simulink model "SMC_Altitude_PID_Position"  (R2021a)
settings: Solver=VariableStepAuto  StartTime=0.0  StopTime=20  RelTol=1e-3
InitFcn:
  | run Quadcopter_setup_parameters.m
values from neighbouring files (symbols this model uses):
  b = 0.001    [Quadcopter_setup_parameters.m]
  Dx = 0.1    [Quadcopter_setup_parameters.m]
  Dy = Dx    (= 0.1)    [Quadcopter_setup_parameters.m]
  Dz = Dx    (= 0.1)    [Quadcopter_setup_parameters.m]
  g = 9.81    [Quadcopter_setup_parameters.m]    (also in recording.mat = 9.80665; uas_parameters.m = 9.80665; uas_parameters.mat = 9.80665)
  I = diag([Ixx; Iyy;Izz],0)    [Quadcopter_setup_parameters.m]
  k = 0.01    [Quadcopter_setup_parameters.m]
  k_phi = 10    [Quadcopter_setup_parameters.m]
  k_psi = 10    [Quadcopter_setup_parameters.m]
  k_theta = 10    [Quadcopter_setup_parameters.m]
  k_z = 10    [Quadcopter_setup_parameters.m]
  kd_xy = 1    [Quadcopter_setup_parameters.m]
  kp_xy = 1    [Quadcopter_setup_parameters.m]
  L = 0.225    [Quadcopter_setup_parameters.m]
  lambda_phi = 2    [Quadcopter_setup_parameters.m]
  lambda_psi = 2    [Quadcopter_setup_parameters.m]
  lambda_theta = 2    [Quadcopter_setup_parameters.m]
  lambda_z = 2    [Quadcopter_setup_parameters.m]
  m = 0.55    [Quadcopter_setup_parameters.m]
settings Model: Creator=Kristian  LastModifiedBy=dwuth
settings SolverCC: AlgebraicLoopSolver=TrustRegion
settings DebuggingCC: SFMachineParentedDataDiag=warning

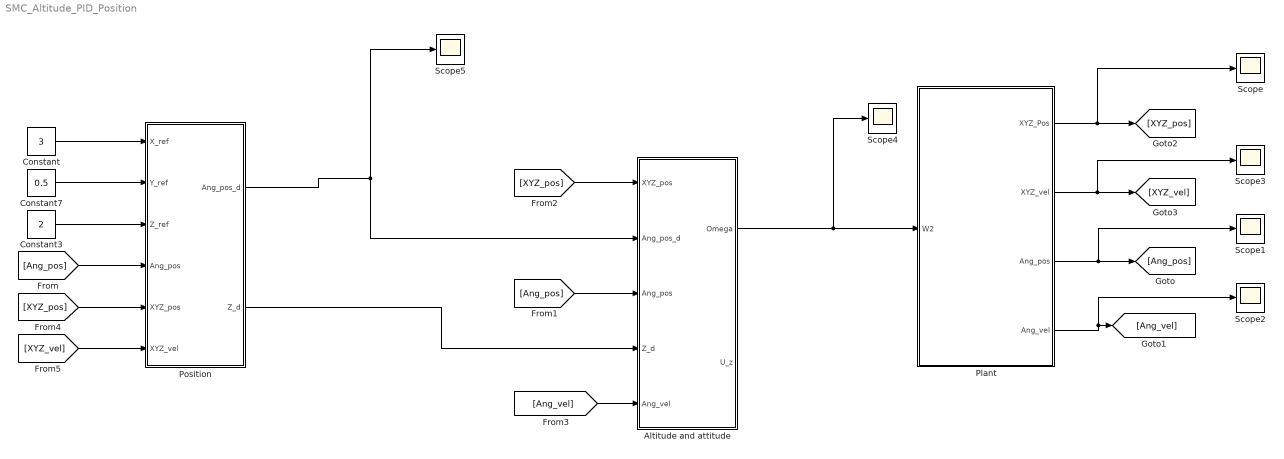
== system SMC_Altitude_PID_Position ==
  Altitude and attitude : Subsystem
  Constant : Constant  Value=3
  Constant3 : Constant  Value=2
  Constant7 : Constant  Value=0.5
  Plant : Subsystem
  Position : Subsystem
  Scope{,1..5} (6 alike) : Scope
  wires:
  Plant/3(Ang_pos) -> [Ang_pos], Scope1/1
  Plant/1(XYZ_Pos) -> [XYZ_pos], Scope/1
  Plant/4(Ang_vel) -> [Ang_vel], Scope2/1
  Altitude and attitude/1(Omega) -> Scope4/1, Plant/1(W2)
  [Ang_vel] -> Altitude and attitude/5(Ang_vel)
  [Ang_pos] -> Altitude and attitude/3(Ang_pos)
  [XYZ_pos] -> Altitude and attitude/1(XYZ_pos)
  Plant/2(XYZ_vel) -> Scope3/1, [XYZ_vel]
  [Ang_pos] -> Position/4(Ang_pos)
  Constant/1 -> Position/1(X_ref)
  Constant7/1 -> Position/2(Y_ref)
  [XYZ_pos] -> Position/5(XYZ_pos)
  [XYZ_vel] -> Position/6(XYZ_vel)
  Position/1(Ang_pos_d) -> Altitude and attitude/2(Ang_pos_d), Scope5/1
  Constant3/1 -> Position/3(Z_ref)
  Position/2(Z_d) -> Altitude and attitude/4(Z_d)

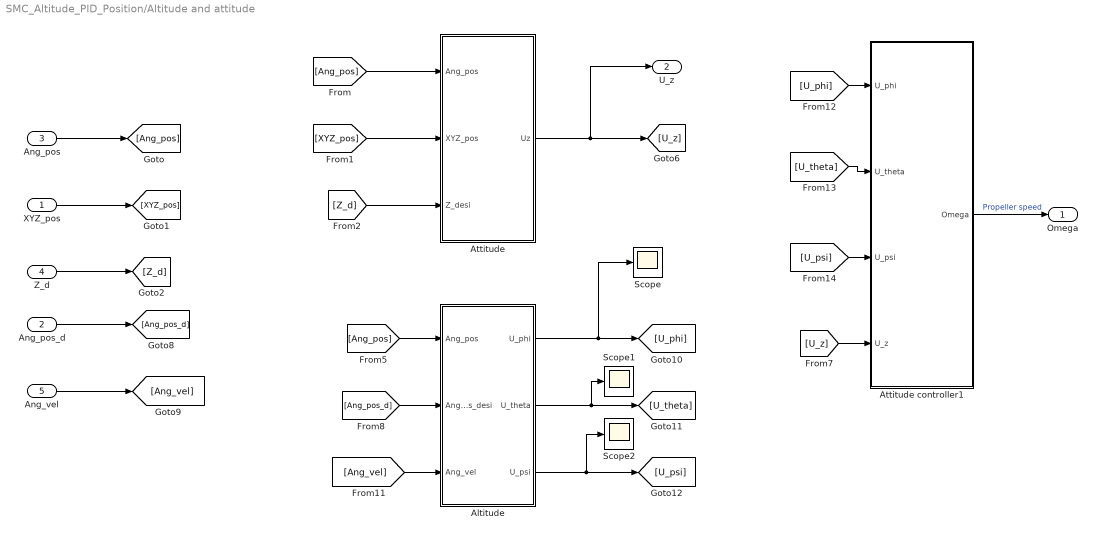
== system SMC_Altitude_PID_Position/Altitude and attitude ==
  XYZ_pos : Inport
  Ang_pos_d : Inport  Port=2
  Ang_pos : Inport  Port=3
  Z_d : Inport  Port=4
  Ang_vel : Inport  Port=5
  Altitude : Subsystem
  Attitude : Subsystem
  Attitude controller1 : MATLAB Function  TreatAsAtomicUnit=on
  Scope : Scope
  Scope1 : Scope
  Scope2 : Scope
  Omega : Outport
  U_z : Outport  Port=2
  wires:
  Attitude controller1/1(Omega) -> Omega/1  "Propeller speed"
  Z_d/1 -> [Z_d]
  [U_theta] -> Attitude controller1/2(U_theta)
  Ang_pos_d/1 -> [Ang_pos_d]
  [XYZ_pos] -> Attitude/2(XYZ_pos)
  Ang_vel/1 -> [Ang_vel]
  [U_phi] -> Attitude controller1/1(U_phi)
  [U_psi] -> Attitude controller1/3(U_psi)
  Ang_pos/1 -> [Ang_pos]
  XYZ_pos/1 -> [XYZ_pos]
  [U_z] -> Attitude controller1/4(U_z)
  [Z_d] -> Attitude/3(Z_desi)
  [Ang_vel] -> Altitude/3(Ang_vel)
  [Ang_pos] -> Altitude/1(Ang_pos)
  [Ang_pos_d] -> Altitude/2(Ang_pos_desi)
  [Ang_pos] -> Attitude/1(Ang_pos)
  Attitude/1(Uz) -> U_z/1, [U_z]
  Altitude/1(U_phi) -> Scope/1, [U_phi]
  Altitude/2(U_theta) -> Scope1/1, [U_theta]
  Altitude/3(U_psi) -> Scope2/1, [U_psi]

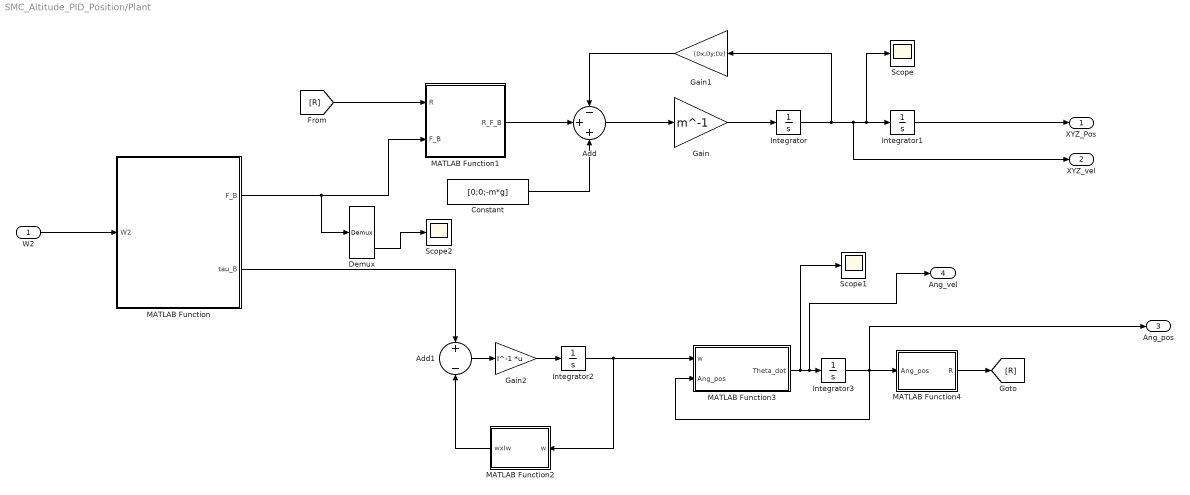
== system SMC_Altitude_PID_Position/Plant ==
  W2 : Inport
  Add : Sum  Inputs=-++
  Add1 : Sum  Inputs=+-
  Constant : Constant  Value=[0;0;-m*g]
  Demux : Demux  Outputs=3
  Gain : Gain  Gain=m^-1
  Gain1 : Gain  Gain=[Dx;Dy;Dz]
  Gain2 : Gain  Gain=I^-1  Multiplication=Matrix(K*u) (u vector)
  Integrator{,1..3} (4 alike) : Integrator
  MATLAB Function : MATLAB Function  TreatAsAtomicUnit=on
  MATLAB Function1 : MATLAB Function  TreatAsAtomicUnit=on
  MATLAB Function2 : MATLAB Function  TreatAsAtomicUnit=on
  MATLAB Function3 : MATLAB Function  TreatAsAtomicUnit=on
  MATLAB Function4 : MATLAB Function  TreatAsAtomicUnit=on
  Scope : Scope
  Scope1 : Scope
  Scope2 : Scope
  XYZ_Pos : Outport
  XYZ_vel : Outport  Port=2
  Ang_pos : Outport  Port=3
  Ang_vel : Outport  Port=4
  wires:
  MATLAB Function/2(tau_B) -> Add1/1
  Gain1/1 -> Add/1
  MATLAB Function/1(F_B) -> Demux/1, MATLAB Function1/2(F_B)
  Gain/1 -> Integrator/1
  MATLAB Function1/1(R_F_B) -> Add/2
  [R] -> MATLAB Function1/1(R)
  Integrator2/1 -> MATLAB Function2/1(w), MATLAB Function3/1(w)
  Gain2/1 -> Integrator2/1
  MATLAB Function2/1(wxIw) -> Add1/2
  Integrator3/1 -> Ang_pos/1, MATLAB Function3/2(Ang_pos), MATLAB Function4/1(Ang_pos)
  Constant/1 -> Add/3
  MATLAB Function3/1(Theta_dot) -> Scope1/1, Ang_vel/1, Integrator3/1
  Add1/1 -> Gain2/1
  Integrator1/1 -> XYZ_Pos/1
  MATLAB Function4/1(R) -> [R]
  Add/1 -> Gain/1
  W2/1 -> MATLAB Function/1(W2)
  Integrator/1 -> Gain1/1, XYZ_vel/1, Scope/1, Integrator1/1
  Demux/3 -> Scope2/1

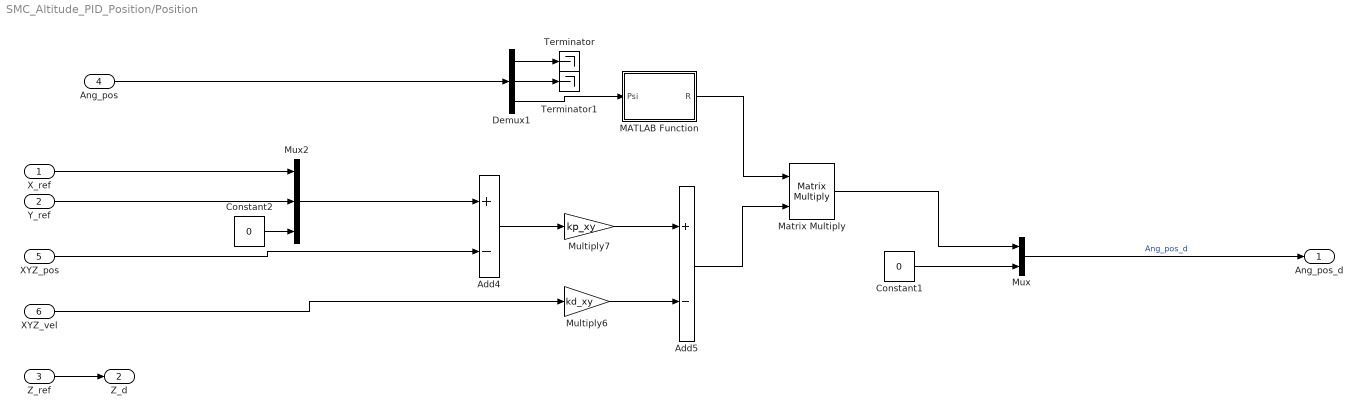
== system SMC_Altitude_PID_Position/Position ==
  X_ref : Inport
  Y_ref : Inport  Port=2
  Z_ref : Inport  Port=3
  Ang_pos : Inport  Port=4
  XYZ_pos : Inport  Port=5
  XYZ_vel : Inport  Port=6
  Add4 : Sum  Inputs=+-
  Add5 : Sum  Inputs=+-
  Constant1 : Constant  Value=0
  Constant2 : Constant  Value=0
  Demux1 : Demux  Outputs=3
  MATLAB Function : MATLAB Function  TreatAsAtomicUnit=on
  Matrix Multiply : Product  Inputs=**  Multiplication=Matrix(*)
  Multiply6 : Gain  Gain=kd_xy
  Multiply7 : Gain  Gain=kp_xy
  Mux : Mux  Inputs=2
  Mux2 : Mux  Inputs=3
  Terminator : Terminator
  Terminator1 : Terminator
  Ang_pos_d : Outport
  Z_d : Outport  Port=2
  wires:
  Matrix Multiply/1 -> Mux/1
  MATLAB Function/1(R) -> Matrix Multiply/1
  Constant2/1 -> Mux2/3
  Mux2/1 -> Add4/1
  Demux1/3 -> MATLAB Function/1(Psi)
  Demux1/1 -> Terminator/1
  Multiply7/1 -> Add5/1
  Demux1/2 -> Terminator1/1
  Add4/1 -> Multiply7/1
  Multiply6/1 -> Add5/2
  Add5/1 -> Matrix Multiply/2
  Constant1/1 -> Mux/2
  XYZ_pos/1 -> Add4/2
  XYZ_vel/1 -> Multiply6/1
  Y_ref/1 -> Mux2/2
  Ang_pos/1 -> Demux1/1
  Mux/1 -> Ang_pos_d/1  "Ang_pos_d"
  X_ref/1 -> Mux2/1
  Z_ref/1 -> Z_d/1

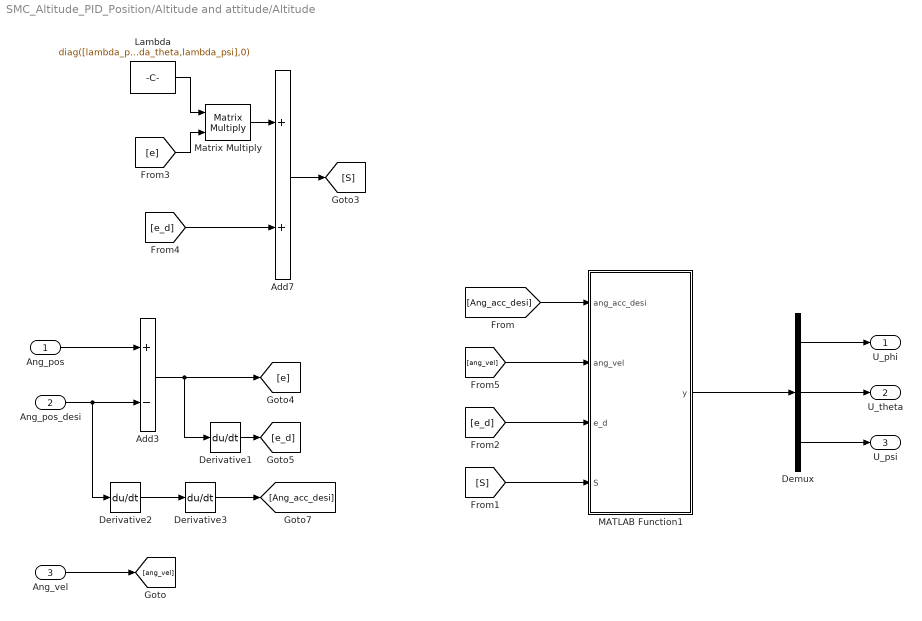
== system SMC_Altitude_PID_Position/Altitude and attitude/Altitude ==
  Ang_pos : Inport
  Ang_pos_desi : Inport  Port=2
  Ang_vel : Inport  Port=3
  Add3 : Sum  Inputs=+-
  Add7 : Sum
  Demux : Demux  Outputs=3
  Derivative1 : Derivative
  Derivative2 : Derivative
  Derivative3 : Derivative
  Lambda : Constant  Value=diag([lambda_phi,lambda_theta,lambda_psi],0)
  MATLAB Function1 : MATLAB Function  TreatAsAtomicUnit=on
  Matrix Multiply : Product  Multiplication=Matrix(*)
  U_phi : Outport
  U_theta : Outport  Port=2
  U_psi : Outport  Port=3
  wires:
  Ang_pos_desi/1 -> Derivative2/1, Add3/2
  [e_d] -> Add7/2
  Derivative1/1 -> [e_d]
  Add7/1 -> [S]
  Add3/1 -> Derivative1/1, [e]
  Derivative3/1 -> [Ang_acc_desi]
  Demux/2 -> U_theta/1
  Derivative2/1 -> Derivative3/1
  Ang_pos/1 -> Add3/1
  Demux/3 -> U_psi/1
  Demux/1 -> U_phi/1
  MATLAB Function1/1(y) -> Demux/1
  [Ang_acc_desi] -> MATLAB Function1/1(ang_acc_desi)
  [e_d] -> MATLAB Function1/3(e_d)
  [S] -> MATLAB Function1/4(S)
  Ang_vel/1 -> [ang_vel]
  [ang_vel] -> MATLAB Function1/2(ang_vel)
  Matrix Multiply/1 -> Add7/1
  [e] -> Matrix Multiply/2
  Lambda/1 -> Matrix Multiply/1

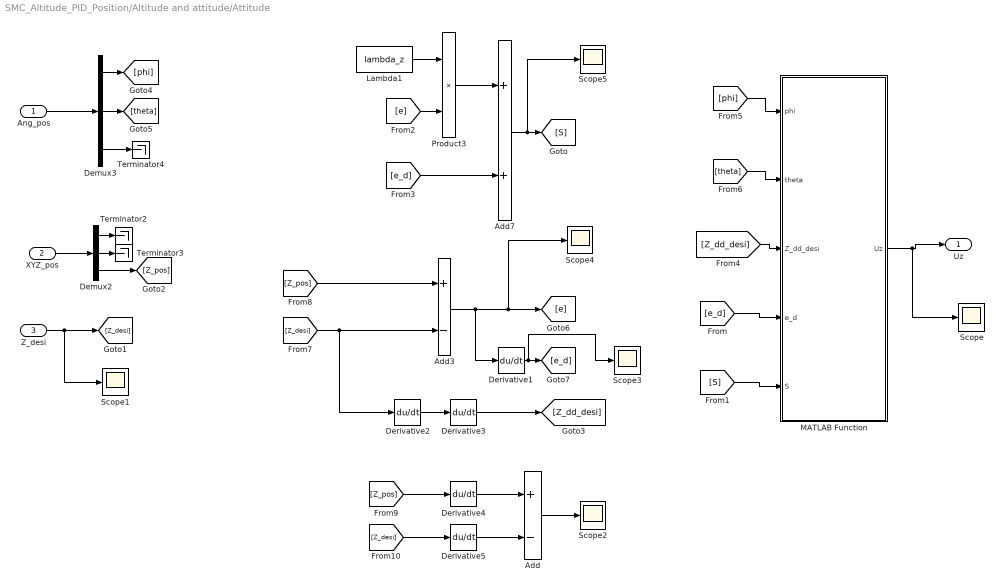
== system SMC_Altitude_PID_Position/Altitude and attitude/Attitude ==
  Ang_pos : Inport
  XYZ_pos : Inport  Port=2
  Z_desi : Inport  Port=3
  Add : Sum  Inputs=+-
  Add3 : Sum  Inputs=+-
  Add7 : Sum
  Demux2 : Demux  Outputs=3
  Demux3 : Demux  Outputs=3
  Derivative{1..5} (5 alike) : Derivative
  Lambda1 : Constant  Value=lambda_z
  MATLAB Function : MATLAB Function  TreatAsAtomicUnit=on
  Product3 : Product
  Scope{,1..5} (6 alike) : Scope
  Terminator2 : Terminator
  Terminator3 : Terminator
  Terminator4 : Terminator
  Uz : Outport
  wires:
  Demux3/2 -> [theta]
  Ang_pos/1 -> Demux3/1
  [theta] -> MATLAB Function/2(theta)
  [Z_dd_desi] -> MATLAB Function/3(Z_dd_desi)
  Add7/1 -> Scope5/1, [S]
  [phi] -> MATLAB Function/1(phi)
  Demux3/3 -> Terminator4/1
  Demux3/1 -> [phi]
  Derivative2/1 -> Derivative3/1
  Derivative3/1 -> [Z_dd_desi]
  Demux2/1 -> Terminator2/1
  Demux2/2 -> Terminator3/1
  [S] -> MATLAB Function/5(S)
  [e] -> Product3/2
  [e_d] -> MATLAB Function/4(e_d)
  Product3/1 -> Add7/1
  [e_d] -> Add7/2
  Lambda1/1 -> Product3/1
  XYZ_pos/1 -> Demux2/1
  MATLAB Function/1(Uz) -> Scope/1, Uz/1
  Add3/1 -> Derivative1/1, Scope4/1, [e]
  Derivative1/1 -> Scope3/1, [e_d]
  Z_desi/1 -> Scope1/1, [Z_desi]
  [Z_desi] -> Derivative2/1, Add3/2
  Demux2/3 -> [Z_pos]
  [Z_pos] -> Add3/1
  [Z_desi] -> Derivative5/1
  [Z_pos] -> Derivative4/1
  Derivative5/1 -> Add/2
  Derivative4/1 -> Add/1
  Add/1 -> Scope2/1

== matlab function SMC_Altitude_PID_Position/Altitude and attitude/Attitude/MATLAB Function ==
  data: phi input; Uz output; theta input; Z_dd_desi input; e_d input; S input; g parameter; m parameter; lambda_z parameter; k_z parameter; k parameter
function Uz = fcn(phi,theta,Z_dd_desi,e_d,S,g, m, lambda_z, k_z,k)

Uz = (m/(k*cos(theta)*cos(phi))) * ( Z_dd_desi + g - lambda_z*e_d-k_z*(2/pi)*atan(100*S) );

== matlab function SMC_Altitude_PID_Position/Altitude and attitude/Attitude controller1 ==
  data: Omega output size=4; U_phi input; U_theta input; U_psi input; U_z input; L parameter; k parameter; b parameter
function Omega = fcn(U_phi, U_theta, U_psi, U_z, L, k, b)

A = [L*k 0 -L*k 0; 0 L*k 0 -L*k; b -b b -b; 1 1 1 1];

U = [U_phi; U_theta; U_psi; U_z];

Omega = (A^-1)*U;

== matlab function SMC_Altitude_PID_Position/Plant/MATLAB Function1 ==
  data: R input; R_F_B output; F_B input
function R_F_B = fcn(R,F_B)

R_F_B = R*F_B;

== matlab function SMC_Altitude_PID_Position/Plant/MATLAB Function ==
  data: W2 input; F_B output; tau_B output; b parameter; k parameter; L parameter
function [F_B, tau_B] = fcn(W2, b, k, L)

F_B = k * [0;0;sum(W2)];

tau_B = [L*k*(W2(1,1)-W2(3,1));
         L*k*(W2(2,1)-W2(4,1))
         b*(W2(1,1)-W2(2,1)+W2(3,1)-W2(4,1))];

== matlab function SMC_Altitude_PID_Position/Plant/MATLAB Function2 ==
  data: w input; wxIw output; I parameter
function wxIw = fcn(w,I)

wxIw = cross(w,(I*w));

== matlab function SMC_Altitude_PID_Position/Plant/MATLAB Function3 ==
  data: w input; Theta_dot output size=3; Ang_pos input
function Theta_dot = fcn(w, Ang_pos)

Phi = Ang_pos(1,1);
Theta = Ang_pos(2,1);
Psi = Ang_pos(3,1);

A = [1 0 -sin(Theta); 0 cos(Psi) cos(Theta)*sin(Phi); 0 -sin(Phi) cos(Theta)*cos(Phi)];

Theta_dot = (A^-1)*w;

== matlab function SMC_Altitude_PID_Position/Plant/MATLAB Function4 ==
  data: Ang_pos input; R output
function R = fcn(Ang_pos)

Phi = Ang_pos(1,1);
Theta = Ang_pos(2,1);
Psi = Ang_pos(3,1);

Rx = [1 0 0; 0 cos(Phi) -sin(Phi); 0 sin(Phi) cos(Phi)];
Ry = [cos(Theta) 0 sin(Theta); 0 1 0; -sin(Theta) 0 cos(Theta)];
Rz = [cos(Psi) -sin(Psi) 0; sin(Psi) cos(Psi) 0; 0 0 1];

R = Rz*Ry*Rx;

== matlab function SMC_Altitude_PID_Position/Position/MATLAB Function ==
  data: Psi input; R output
function R = fcn(Psi)

R = [sin(Psi) -cos(Psi) 0;cos(Psi) sin(Psi) 0];

== matlab function SMC_Altitude_PID_Position/Altitude and attitude/Altitude/MATLAB Function1 ==
  data: y output; ang_acc_desi input; ang_vel input; e_d input; S input; I parameter; lambda_phi parameter; lambda_theta parameter; lambda_psi parameter; k_phi parameter; k_theta parameter; k_psi parameter
function y = fcn(ang_acc_desi, ang_vel, e_d,S, I, lambda_phi, lambda_theta, lambda_psi, k_phi, k_theta, k_psi)

lambda = [lambda_phi 0 0; 0 lambda_theta 0; 0 0 lambda_psi];
k = diag([k_phi;k_theta;k_psi],0);
%I = [Ixx 0 0; 0 Iyy 0; 0 0 Izz];
I_extra = diag([(I(2,2)-I(3,3));(I(3,3)-I(1,1));I(1,1)-I(2,2)],0);
ang_vel_extra = [ang_vel(2)*ang_vel(3);ang_vel(1)*ang_vel(3);ang_vel(1)*ang_vel(2)];

y = I *(ang_acc_desi + lambda*e_d - k*(2/pi)*atan(100*S)) - I_extra*ang_vel_extra;
